simulink model "S_MPPT_ALGS_PIL_SIM_V1"  (R2017a)
settings: Solver=VariableStepAuto  StartTime=0.0  StopTime=5  FixedStep=1e-6  MaxStep=1e-4  RelTol=1e-3
values from neighbouring files (symbols this model uses):
  Alpha1 = 2*Zeta_obs*wn_obs    (= 2)    [M_MPPT_ALGS_PIL_SIM_V1.m]
  Alpha2 = wn_obs    (= 1)    [M_MPPT_ALGS_PIL_SIM_V1.m]
  Cdc = Cdc    (= 0.00047)    [M_MPPT_ALGS_PIL_SIM_V1.m]
  Cpv = Cpv    (= 8e-05)    [M_MPPT_ALGS_PIL_SIM_V1.m]
  Epsilon = Ep_cont/Ts1    [M_MPPT_ALGS_PIL_SIM_V1.m]
  ESRCdc = ESRCdc    (= 0.2)    [M_MPPT_ALGS_PIL_SIM_V1.m]
  ESRCpv = ESRCpv    (= 0.2)    [M_MPPT_ALGS_PIL_SIM_V1.m]
  Fred = fs    (= 60)    [M_MPPT_ALGS_PIL_SIM_V1.m]
  fs = 60    [M_MPPT_ALGS_PIL_SIM_V1.m]
  G_STC = 1000    [M_MPPT_ALGS_PIL_SIM_V1.m]
  Icc_calc = In/(5/100)    [M_MPPT_ALGS_PIL_SIM_V1.m]
  impp_STC = 15.72/2    (= 7.86)    [M_MPPT_ALGS_PIL_SIM_V1.m]
  K1 = Kt_acker_d    [M_MPPT_ALGS_PIL_SIM_V1.m]
  K1y2md = Kmd(1:end-1)    [M_MPPT_ALGS_PIL_SIM_V1.m]
  Kdpwm = 1/Ucmax    (= 1.52590218967e-05)    [M_MPPT_ALGS_PIL_SIM_V1.m]
  KI1 = Kp1/Ti1*Ts1    (= 1900)    [M_MPPT_ALGS_PIL_SIM_V1.m]
  KI2 = Ki2*Ts4    [M_MPPT_ALGS_PIL_SIM_V1.m]
  KI4 = Ki4*Ts4    [M_MPPT_ALGS_PIL_SIM_V1.m]
  KI5 = Ki5*Ts_inv    (= 0.17765287922)    [M_MPPT_ALGS_PIL_SIM_V1.m]
  Kimd = -Kmd(end)    [M_MPPT_ALGS_PIL_SIM_V1.m]
  KP1 = Kp1-KI1/2    (= 21850)    [M_MPPT_ALGS_PIL_SIM_V1.m]
  KP2 = Kp2-KI2/2    [M_MPPT_ALGS_PIL_SIM_V1.m]
  KP4 = Kp4-KI4/2    [M_MPPT_ALGS_PIL_SIM_V1.m]
  KP5 = Kp5*Ts_inv-KI5/2    (= -0.0874937760062)    [M_MPPT_ALGS_PIL_SIM_V1.m]
  L = L    (= 0.1)    [M_MPPT_ALGS_PIL_SIM_V1.m]
  Linv = 0.03    [M_MPPT_ALGS_PIL_SIM_V1.m]
  Npar = No_Cadenas_Paralelo    (= 2)    [M_MPPT_ALGS_PIL_SIM_V1.m]
  Rinv = 0.0417    [M_MPPT_ALGS_PIL_SIM_V1.m]
  RL = RL    (= 0.3)    [M_MPPT_ALGS_PIL_SIM_V1.m]
  S = 10e3*3/2    (= 15000)    [M_MPPT_ALGS_PIL_SIM_V1.m]
  Ts = Ts1    (= 0.0002)    [M_MPPT_ALGS_PIL_SIM_V1.m]
  Ts1 = 1/Fs    (= 0.0002)    [M_MPPT_ALGS_PIL_SIM_V1.m]
  Ts4 = 1/(4*Fc)    (= 0.000125)    [M_MPPT_ALGS_PIL_SIM_V1.m]
  Ts_inv = 1/(100*Fc)    (= 5e-06)    [M_MPPT_ALGS_PIL_SIM_V1.m]
  Ucmax = (2^b-1)    (= 65535)    [M_MPPT_ALGS_PIL_SIM_V1.m]
  vdc = 1000    [M_MPPT_ALGS_PIL_SIM_V1.m]
  vdc_ref = vdc    (= 1000)    [M_MPPT_ALGS_PIL_SIM_V1.m]
  Vf = VL/sqrt(3)    [M_MPPT_ALGS_PIL_SIM_V1.m]
  VL = (381.051/2)    (= 190.5255)    [M_MPPT_ALGS_PIL_SIM_V1.m]
undefined symbols (not defined in the file or in its folder): DiscIntNeverNeededParam
undefined symbols (not defined in the file): Fs
libraries: powerlib x15, powerlib_meascontrol x12, dsparch4 x3, re_lib x1
(part 2 of 2)

== matlab function S_MPPT_ALGS_PIL_SIM_V1/B Measumerents/Subsystem3/MATLAB Function ==
  data: uc_avg output; uc input; time input; t_start input; t_end input
function uc_avg = control_effort_avg(uc, time, t_start, t_end)
%#codegen
% Calcula el valor promedio acumulado del esfuerzo de control
% solo dentro del intervalo [t_start, t_end].
%
% Entradas:
%   uc      : señal de control instantánea (ej. ciclo de trabajo o voltaje)
%   time    : tiempo actual (segundos)
%   t_start : tiempo desde el cual se comienza a acumular
%   t_end   : tiempo en el que se detiene la acumulación
%
% Salida:
%   uc_avg : valor promedio acumulado del esfuerzo de control

% Variables persistentes
persistent sum_u sample_count started

% Inicialización
if isempty(sum_u)
    sum_u = 0;
    sample_count = 0;
    started = false;
end

% Acumulación solo dentro del intervalo [t_start, t_end]
if time >= t_start && time <= t_end
    if ~started
        started = true; % se activa solo la primera vez que entra al intervalo
    end

    sum_u = sum_u + abs(uc); % acumulación del valor absoluto
    sample_count = sample_count + 1;
end

% Cálculo del promedio acumulado
if sample_count == 0
    uc_avg = 0;
else
    uc_avg = sum_u / sample_count;
end
end

== matlab function S_MPPT_ALGS_PIL_SIM_V1/B Measumerents/Subsystem4/MATLAB Function ==
  data: uc_avg output; uc input; time input; t_start input; t_end input
function uc_avg = control_effort_avg(uc, time, t_start, t_end)
%#codegen
% Calcula el valor promedio acumulado del esfuerzo de control
% solo dentro del intervalo [t_start, t_end].
%
% Entradas:
%   uc      : señal de control instantánea (ej. ciclo de trabajo o voltaje)
%   time    : tiempo actual (segundos)
%   t_start : tiempo desde el cual se comienza a acumular
%   t_end   : tiempo en el que se detiene la acumulación
%
% Salida:
%   uc_avg : valor promedio acumulado del esfuerzo de control

% Variables persistentes
persistent sum_u sample_count started

% Inicialización
if isempty(sum_u)
    sum_u = 0;
    sample_count = 0;
    started = false;
end

% Acumulación solo dentro del intervalo [t_start, t_end]
if time >= t_start && time <= t_end
    if ~started
        started = true; % se activa solo la primera vez que entra al intervalo
    end

    sum_u = sum_u + abs(uc); % acumulación del valor absoluto
    sample_count = sample_count + 1;
end

% Cálculo del promedio acumulado
if sample_count == 0
    uc_avg = 0;
else
    uc_avg = sum_u / sample_count;
end
end

== matlab function S_MPPT_ALGS_PIL_SIM_V1/B Measumerents/Subsystem6/MATLAB Function ==
  data: ah output; current input; time input; t_start input; t_end input; i_avg output
function [ah, i_avg] = ah_accumulator(current, time, t_start, t_end)
%#codegen
% Calcula la carga acumulada en Ah y la corriente promedio en el intervalo [t_start, t_end]

% Entradas:
%   current : corriente instantánea (A)
%   time    : tiempo actual (s)
%   t_start : tiempo de inicio del intervalo (s)
%   t_end   : tiempo de fin del intervalo (s)
%
% Salidas:
%   ah    : carga acumulada en Ah
%   i_avg : corriente promedio (A)

% Variables persistentes
persistent last_time total_Ah started current_sum sample_count

% Inicialización al primer uso
if isempty(total_Ah)
    total_Ah = 0;
    last_time = 0;
    started = false;
    current_sum = 0;
    sample_count = 0;
end

% Solo acumular si dentro del intervalo
if time >= t_start && time <= t_end
    if ~started
        last_time = time;
        started = true;
    end

    dt = time - last_time;
    if dt > 0
        total_Ah = total_Ah + (current * dt) / 3600;
        last_time = time;
    end

    % Acumular para promedio
    current_sum = current_sum + current;
    sample_count = sample_count + 1;
end

% Resultados
ah = total_Ah;

% Corriente promedio solo si hay muestras válidas
if sample_count > 0
    i_avg = current_sum / sample_count;
else
    i_avg = 0;
end
end

== matlab function S_MPPT_ALGS_PIL_SIM_V1/B Measumerents/Subsystem7/MATLAB Function ==
  data: ah output; current input; time input; t_start input; t_end input; i_avg output
function [ah, i_avg] = ah_accumulator(current, time, t_start, t_end)
%#codegen
% Calcula la carga acumulada en Ah y la corriente promedio en el intervalo [t_start, t_end]

% Entradas:
%   current : corriente instantánea (A)
%   time    : tiempo actual (s)
%   t_start : tiempo de inicio del intervalo (s)
%   t_end   : tiempo de fin del intervalo (s)
%
% Salidas:
%   ah    : carga acumulada en Ah
%   i_avg : corriente promedio (A)

% Variables persistentes
persistent last_time total_Ah started current_sum sample_count

% Inicialización al primer uso
if isempty(total_Ah)
    total_Ah = 0;
    last_time = 0;
    started = false;
    current_sum = 0;
    sample_count = 0;
end

% Solo acumular si dentro del intervalo
if time >= t_start && time <= t_end
    if ~started
        last_time = time;
        started = true;
    end

    dt = time - last_time;
    if dt > 0
        total_Ah = total_Ah + (current * dt) / 3600;
        last_time = time;
    end

    % Acumular para promedio
    current_sum = current_sum + current;
    sample_count = sample_count + 1;
end

% Resultados
ah = total_Ah;

% Corriente promedio solo si hay muestras válidas
if sample_count > 0
    i_avg = current_sum / sample_count;
else
    i_avg = 0;
end
end

== matlab function S_MPPT_ALGS_PIL_SIM_V1/B Measumerents/Subsystem8/MATLAB Function ==
  data: energy_wh output; power_kw input; time input; t_start input; t_end input; power_avg output
function [energy_wh, power_avg] = wh_accumulator(power_kw, time, t_start, t_end)
%#codegen
% Calcula la energía acumulada (Wh) y potencia promedio (kW)
% dentro del intervalo de tiempo [t_start, t_end].

% Entradas:
%   power_kw : potencia instantánea en kilowatts (kW)
%   time     : tiempo actual (s)
%   t_start  : tiempo inicial (s)
%   t_end    : tiempo final (s)
%
% Salidas:
%   energy_wh : energía acumulada en Wh
%   power_avg : potencia promedio en kW

% Variables persistentes
persistent last_time total_energy_wh started sum_power sample_count

% Inicialización al primer uso
if isempty(total_energy_wh)
    total_energy_wh = 0;
    last_time = 0;
    started = false;
    sum_power = 0;
    sample_count = 0;
end

% Solo acumular si dentro del intervalo
if time >= t_start && time <= t_end
    if ~started
        last_time = time;
        started = true;
    end

    dt = time - last_time;
    if dt > 0
        % Energía en Wh: P(kW) * dt (s) * (1000 / 3600)
        total_energy_wh = total_energy_wh + (power_kw * dt) * (1000 / 3600);
        last_time = time;
    end

    % Para el promedio de potencia
    sum_power = sum_power + power_kw;
    sample_count = sample_count + 1;
end

% Salidas
energy_wh = total_energy_wh;

if sample_count > 0
    power_avg = 1000*(sum_power / sample_count);
else
    power_avg = 0;
end
end

== matlab function S_MPPT_ALGS_PIL_SIM_V1/B Measumerents/Subsystem9/MATLAB Function ==
  data: energy_wh output; power_kw input; time input; t_start input; t_end input; power_avg output
function [energy_wh, power_avg] = wh_accumulator(power_kw, time, t_start, t_end)
%#codegen
% Calcula la energía acumulada (Wh) y potencia promedio (kW)
% dentro del intervalo de tiempo [t_start, t_end].

% Entradas:
%   power_kw : potencia instantánea en kilowatts (kW)
%   time     : tiempo actual (s)
%   t_start  : tiempo inicial (s)
%   t_end    : tiempo final (s)
%
% Salidas:
%   energy_wh : energía acumulada en Wh
%   power_avg : potencia promedio en kW

% Variables persistentes
persistent last_time total_energy_wh started sum_power sample_count

% Inicialización al primer uso
if isempty(total_energy_wh)
    total_energy_wh = 0;
    last_time = 0;
    started = false;
    sum_power = 0;
    sample_count = 0;
end

% Solo acumular si dentro del intervalo
if time >= t_start && time <= t_end
    if ~started
        last_time = time;
        started = true;
    end

    dt = time - last_time;
    if dt > 0
        % Energía en Wh: P(kW) * dt (s) * (1000 / 3600)
        total_energy_wh = total_energy_wh + (power_kw * dt) * (1000 / 3600);
        last_time = time;
    end

    % Para el promedio de potencia
    sum_power = sum_power + power_kw;
    sample_count = sample_count + 1;
end

% Salidas
energy_wh = total_energy_wh;

if sample_count > 0
    power_avg = 1000*(sum_power / sample_count);
else
    power_avg = 0;
end
end

== matlab function S_MPPT_ALGS_PIL_SIM_V1/B Measumerents/Subsystem10/MATLAB Function ==
  data: ah output; current input; time input; t_start input; t_end input; i_avg output
function [ah, i_avg] = ah_accumulator(current, time, t_start, t_end)
%#codegen
% Calcula la carga acumulada en Ah y la corriente promedio en el intervalo [t_start, t_end]

% Entradas:
%   current : corriente instantánea (A)
%   time    : tiempo actual (s)
%   t_start : tiempo de inicio del intervalo (s)
%   t_end   : tiempo de fin del intervalo (s)
%
% Salidas:
%   ah    : carga acumulada en Ah
%   i_avg : corriente promedio (A)

% Variables persistentes
persistent last_time total_Ah started current_sum sample_count

% Inicialización al primer uso
if isempty(total_Ah)
    total_Ah = 0;
    last_time = 0;
    started = false;
    current_sum = 0;
    sample_count = 0;
end

% Solo acumular si dentro del intervalo
if time >= t_start && time <= t_end
    if ~started
        last_time = time;
        started = true;
    end

    dt = time - last_time;
    if dt > 0
        total_Ah = total_Ah + (current * dt) / 3600;
        last_time = time;
    end

    % Acumular para promedio
    current_sum = current_sum + current;
    sample_count = sample_count + 1;
end

% Resultados
ah = total_Ah;

% Corriente promedio solo si hay muestras válidas
if sample_count > 0
    i_avg = current_sum / sample_count;
else
    i_avg = 0;
end
end

== matlab function S_MPPT_ALGS_PIL_SIM_V1/B Measumerents/Subsystem11/MATLAB Function ==
  data: uc_avg output; uc input; time input; t_start input; t_end input
function uc_avg = control_effort_avg(uc, time, t_start, t_end)
%#codegen
% Calcula el valor promedio acumulado del esfuerzo de control
% solo dentro del intervalo [t_start, t_end].
%
% Entradas:
%   uc      : señal de control instantánea (ej. ciclo de trabajo o voltaje)
%   time    : tiempo actual (segundos)
%   t_start : tiempo desde el cual se comienza a acumular
%   t_end   : tiempo en el que se detiene la acumulación
%
% Salida:
%   uc_avg : valor promedio acumulado del esfuerzo de control

% Variables persistentes
persistent sum_u sample_count started

% Inicialización
if isempty(sum_u)
    sum_u = 0;
    sample_count = 0;
    started = false;
end

% Acumulación solo dentro del intervalo [t_start, t_end]
if time >= t_start && time <= t_end
    if ~started
        started = true; % se activa solo la primera vez que entra al intervalo
    end

    sum_u = sum_u + abs(uc); % acumulación del valor absoluto
    sample_count = sample_count + 1;
end

% Cálculo del promedio acumulado
if sample_count == 0
    uc_avg = 0;
else
    uc_avg = sum_u / sample_count;
end
end

== matlab function S_MPPT_ALGS_PIL_SIM_V1/B Measumerents/Subsystem12/MATLAB Function ==
  data: efficiency output; Pmpp input; Pactual input; time input; t_start input; t_end input

function efficiency = n_mppt(Pmpp, Pactual, time, t_start, t_end)
%#codegen
% Calcula la eficiencia acumulada de un MPPT en porcentaje
% limitando Pactual para que no exceda Pmpp.
% Acumula solo dentro del intervalo de tiempo [t_start, t_end].
%
% Entradas:
%   Pmpp     : potencia teórica máxima (kW)
%   Pactual  : potencia medida real (kW)
%   time     : tiempo actual (segundos)
%   t_start  : inicio de acumulación
%   t_end    : fin de acumulación
%
% Salida:
%   efficiency : eficiencia acumulada (%), limitada a 100

% Variables persistentes
persistent total_Pmpp total_Pactual started

% Inicialización al primer uso
if isempty(total_Pmpp)
    total_Pmpp = 0;
    total_Pactual = 0;
    started = false;
end

% Acumular solo dentro del intervalo [t_start, t_end]
if time >= t_start && time <= t_end
    if ~started
        started = true;
    end

    % Limitar Pactual para evitar que exceda Pmpp
    %Pactual_limited = min(Pactual, Pmpp);
     
    % No Limitar Pactual 
    Pactual_limited = Pactual;

    % Acumulación
    total_Pmpp = total_Pmpp + Pmpp;
    total_Pactual = total_Pactual + Pactual_limited;
end

% Cálculo de eficiencia acumulada
if total_Pmpp < 1e-6
    efficiency = 0;
else
    efficiency = min((total_Pactual / total_Pmpp) * 100, 100);
end
end

== matlab function S_MPPT_ALGS_PIL_SIM_V1/B Measumerents/Subsystem14/MATLAB Function ==
  data: energy_wh output; power_kw input; time input; t_start input; t_end input; power_avg output
function [energy_wh, power_avg] = wh_accumulator(power_kw, time, t_start, t_end)
%#codegen
% Calcula la energía acumulada (Wh) y potencia promedio (kW)
% dentro del intervalo de tiempo [t_start, t_end].

% Entradas:
%   power_kw : potencia instantánea en kilowatts (kW)
%   time     : tiempo actual (s)
%   t_start  : tiempo inicial (s)
%   t_end    : tiempo final (s)
%
% Salidas:
%   energy_wh : energía acumulada en Wh
%   power_avg : potencia promedio en kW

% Variables persistentes
persistent last_time total_energy_wh started sum_power sample_count

% Inicialización al primer uso
if isempty(total_energy_wh)
    total_energy_wh = 0;
    last_time = 0;
    started = false;
    sum_power = 0;
    sample_count = 0;
end

% Solo acumular si dentro del intervalo
if time >= t_start && time <= t_end
    if ~started
        last_time = time;
        started = true;
    end

    dt = time - last_time;
    if dt > 0
        % Energía en Wh: P(kW) * dt (s) * (1000 / 3600)
        total_energy_wh = total_energy_wh + (power_kw * dt) * (1000 / 3600);
        last_time = time;
    end

    % Para el promedio de potencia
    sum_power = sum_power + power_kw;
    sample_count = sample_count + 1;
end

% Salidas
energy_wh = total_energy_wh;

if sample_count > 0
    power_avg = 1000*(sum_power / sample_count);
else
    power_avg = 0;
end
end
